simulink library "First_Order_Filter_lib"  (Simulink 7.2)
settings: Solver=ode45  SolverMode=SingleTasking  StartTime=0.0  StopTime=10.0  RelTol=1e-3
undefined symbols (not defined in the file or in its folder): DiscIntNeverNeededParam, POS_hi, POS_lo, Timestep
libraries: simulink x1
settings Model: Creator=cbuttril  LastModifiedBy=amurch

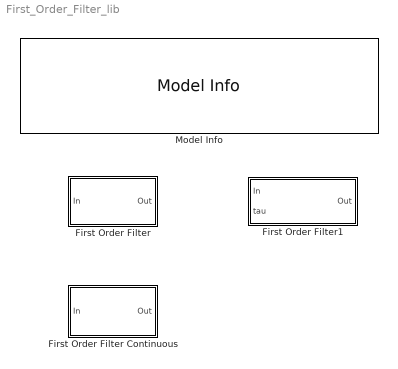
== system First_Order_Filter_lib ==
  First Order Filter : Subsystem  mask(first order filter){tau=0.1, timestep=Timestep}
      mask help:
      | __1__
      |  tau s+1
      |
      | First order filter  transfer function
      | with integrator IC = input  at time=0
      | If tau < Simulation Timestep, input is passed through unchanged
      | Simulation timestep must be a variable in the model/base workspace named
      | "Timestep"
      mask Help:
      | This block models a first order filter with the initial condition
      | on the integrator set to the steady state value for constant input.
      | time constant is an input
      mask Display: fprintf('  1\n--------------\n %2.1g s + 1', tau)
  First Order Filter Continuous : Subsystem  mask(first order filter){tau=0.1}
      mask help:
      | __1__
      |  tau s+1
      |
      | First order filter  transfer function
      | with integrator IC = input  at time=0
      |
      | Uses continuous time integrator.
      mask Display: fprintf('  1\n--------------\n %2.1g s + 1', tau)
  First Order Filter1 : Subsystem  mask(first order filter){timestep=Timestep}
      mask help:
      | __1__
      |  tau s+1
      |
      | First order filter  transfer function
      | with integrator IC = input  at time=0
      | If tau < Simulation Timestep, input is passed through unchanged
      mask Help:
      | This block models a first order filter with the initial condition
      | on the integrator set to the steady state value for constant input.
      | time constant is an input
      mask Display:
      | fprintf('  1\n________\ntau * s + 1')
      | 
      | port_label('input',1,'signal')
      | port_label('input',2,'tau')
  Model Info : simulink/Model-Wide Utilities/Model Info  SystemSampleTime=-1  InitialBlockCM=None  BlockCM=None  Frame=on  DisplayStringWithTags=|  HorizontalTextAlignment=Center  LeftAlignmentValue=0.5  SourceBlockDiagram=First_Order_Filter_lib  TagMaxNumber=20
      | Developed using Matlab Release 2007a
      | 
      | SVN:%<ModelVersion>
      | Last modifed by %<LastModifiedBy> on %<LastModificationDate>

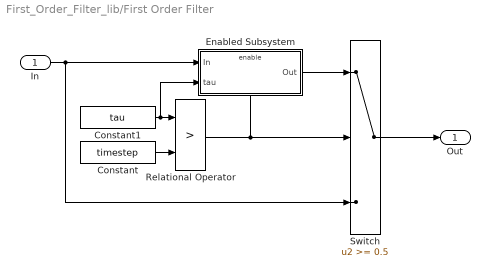
== system First_Order_Filter_lib/First Order Filter ==
  In : Inport  OutDataType=sfix(16)  OutScaling=2^0
  Constant : Constant  Value=timestep  OutDataType=sfix(16)  OutScaling=2^0
  Constant1 : Constant  Value=tau  OutDataType=sfix(16)  OutScaling=2^0
  Enabled Subsystem : Subsystem  TreatAsAtomicUnit=on
  Relational Operator : RelationalOperator  Operator=>  LogicOutDataTypeMode=boolean  OutDataTypeStr=boolean
  Switch : Switch  Threshold=0.5  SampleTime=Timestep
  Out : Outport  OutDataType=sfix(16)  OutScaling=2^0
  wires:
  Constant1/1 -> Enabled Subsystem/2(tau), Relational Operator/1
  Enabled Subsystem/1(Out) -> Switch/1
  Switch/1 -> Out/1
  In/1 -> Enabled Subsystem/1(In), Switch/3
  Relational Operator/1 -> Enabled Subsystem/Enable, Switch/2
  Constant/1 -> Relational Operator/2

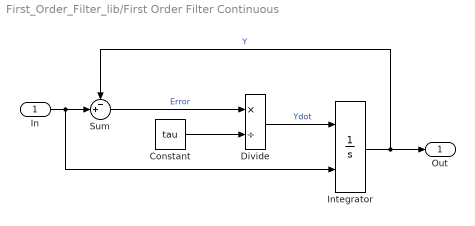
== system First_Order_Filter_lib/First Order Filter Continuous ==
  In : Inport  OutDataType=sfix(16)  OutScaling=2^0
  Constant : Constant  Value=tau  OutDataType=sfix(16)  OutScaling=2^0
  Divide : Product  Inputs=*/  OutDataType=sfix(16)  OutScaling=2^-10
  Integrator : Integrator  InitialConditionSource=external
  Sum : Sum  Inputs=-+|  OutDataType=sfix(16)  OutScaling=2^0  SaturateOnIntegerOverflow=on  InputSameDT=on  OutDataTypeStr=Inherit: Same as first input
  Out : Outport  OutDataType=sfix(16)  OutScaling=2^0
  wires:
  Divide/1 -> Integrator/1  "Ydot"
  Integrator/1 -> Sum/1, Out/1  "Y"
  In/1 -> Sum/2, Integrator/2
  Sum/1 -> Divide/1  "Error"
  Constant/1 -> Divide/2

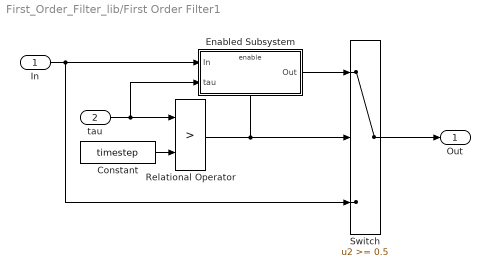
== system First_Order_Filter_lib/First Order Filter1 ==
  In : Inport  OutDataType=sfix(16)  OutScaling=2^0
  tau : Inport  Port=2  OutDataType=sfix(16)  OutScaling=2^0
  Constant : Constant  Value=timestep  OutDataType=sfix(16)  OutScaling=2^0
  Enabled Subsystem : Subsystem  TreatAsAtomicUnit=on
  Relational Operator : RelationalOperator  Operator=>  LogicOutDataTypeMode=boolean  OutDataTypeStr=boolean
  Switch : Switch  Threshold=0.5  SampleTime=Timestep
  Out : Outport  OutDataType=sfix(16)  OutScaling=2^0
  wires:
  Constant/1 -> Relational Operator/2
  Relational Operator/1 -> Switch/2, Enabled Subsystem/Enable
  In/1 -> Switch/3, Enabled Subsystem/1(In)
  tau/1 -> Relational Operator/1, Enabled Subsystem/2(tau)
  Switch/1 -> Out/1
  Enabled Subsystem/1(Out) -> Switch/1

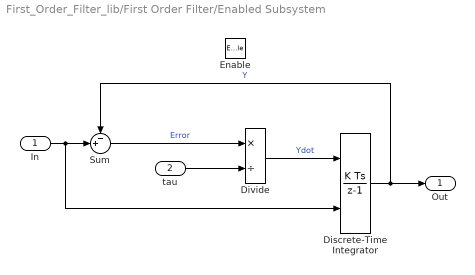
== system First_Order_Filter_lib/First Order Filter/Enabled Subsystem ==
  In : Inport  OutDataType=sfix(16)  OutScaling=2^0
  tau : Inport  Port=2  OutDataType=sfix(16)  OutScaling=2^0
  Enable : EnablePort  StatesWhenEnabling=reset
  Discrete-Time Integrator : DiscreteIntegrator  InitialConditionSource=external  SampleTime=Timestep  OutDataType=sfix(16)  OutScaling=2^0  ICPrevOutput=DiscIntNeverNeededParam  ICPrevScaledInput=DiscIntNeverNeededParam
  Divide : Product  Inputs=*/  OutDataType=sfix(16)  OutScaling=2^-10
  Sum : Sum  Inputs=-+|  OutDataType=sfix(16)  OutScaling=2^0  SaturateOnIntegerOverflow=on  InputSameDT=on  OutDataTypeStr=Inherit: Same as first input
  Out : Outport  OutDataType=sfix(16)  OutScaling=2^0
  wires:
  Sum/1 -> Divide/1  "Error"
  In/1 -> Discrete-Time Integrator/2, Sum/2
  Discrete-Time Integrator/1 -> Out/1, Sum/1  "Y"
  tau/1 -> Divide/2
  Divide/1 -> Discrete-Time Integrator/1  "Ydot"

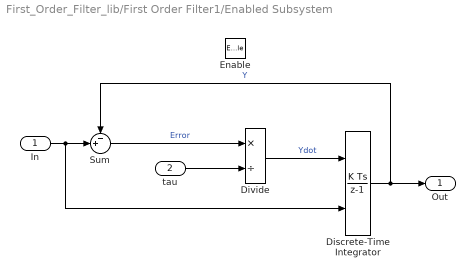
== system First_Order_Filter_lib/First Order Filter1/Enabled Subsystem ==
  In : Inport  OutDataType=sfix(16)  OutScaling=2^0
  tau : Inport  Port=2  OutDataType=sfix(16)  OutScaling=2^0
  Enable : EnablePort
  Discrete-Time Integrator : DiscreteIntegrator  InitialConditionSource=external  SampleTime=Timestep  OutDataType=sfix(16)  OutScaling=2^0  UpperSaturationLimit=POS_hi  LowerSaturationLimit=POS_lo  ICPrevOutput=DiscIntNeverNeededParam  ICPrevScaledInput=DiscIntNeverNeededParam
  Divide : Product  Inputs=*/  OutDataType=sfix(16)  OutScaling=2^-10
  Sum : Sum  Inputs=-+|  OutDataType=sfix(16)  OutScaling=2^0  SaturateOnIntegerOverflow=on  InputSameDT=on  OutDataTypeStr=Inherit: Same as first input
  Out : Outport  OutDataType=sfix(16)  OutScaling=2^0
  wires:
  Divide/1 -> Discrete-Time Integrator/1  "Ydot"
  tau/1 -> Divide/2
  Discrete-Time Integrator/1 -> Sum/1, Out/1  "Y"
  In/1 -> Discrete-Time Integrator/2, Sum/2
  Sum/1 -> Divide/1  "Error"
